simulink model "switchcase"  (R2024a)
settings: Solver=FixedStepAuto  StartTime=0.0  StopTime=10.0  FixedStep=0.5  RelTol=1e-3
settings Model: Creator=DELL  LastModifiedBy=DELL

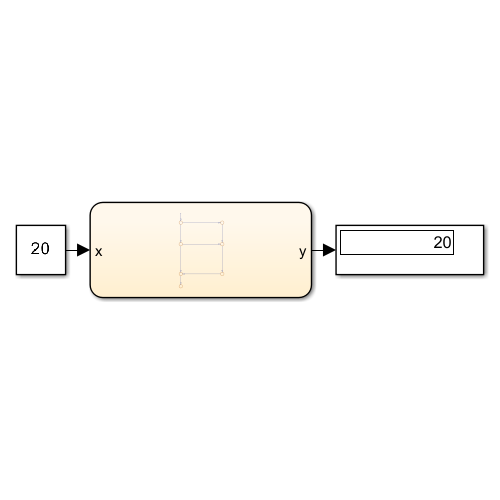
[thumbnail: Simulink's stored preview of the top-level diagram]
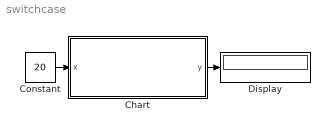
== system switchcase ==
  Chart : Stateflow chart  TreatAsAtomicUnit=on
  Constant : Constant  Value=20
  Display : Display
  wires:
  Constant/1 -> Chart/1(x)
  Chart/1(y) -> Display/1

== stateflow chart switchcase/Chart ==
  note: /*if condition */
  note: /*if action*/
  note: /*elif condition */
  note: /*if action*/
  note: /*else action */
  note: /*terminate point */
  (default) -> (junction 35)
  (junction 35) -> (junction 39) [order 1] : [x==0]
  (junction 35) -> (junction 54) [order 2]
  (junction 39) -> (junction 55) : {y++}
  (junction 54) -> (junction 55) [order 1] : [x==20]
  (junction 54) -> (junction 45) [order 2] : {y--}
  (junction 55) -> (junction 38) : {y=20}
  (junction 38) -> (junction 45)
  (junction 45) -> (junction 46)
  data: x input; y output double =1
